simulink library "gps_block_visual"  (R2025b)
settings: Solver=VariableStepAuto  StartTime=0.0  StopTime=10.0  RelTol=1e-3
values from neighbouring files (symbols this model uses):
  GPS = evalin('base', 'GPS')    [test_gps_model.m]
  Sim = evalin('base', 'Sim')    [test_gps_model.m]
settings Model: Creator=Ashwin  LastModifiedBy=Ashwin

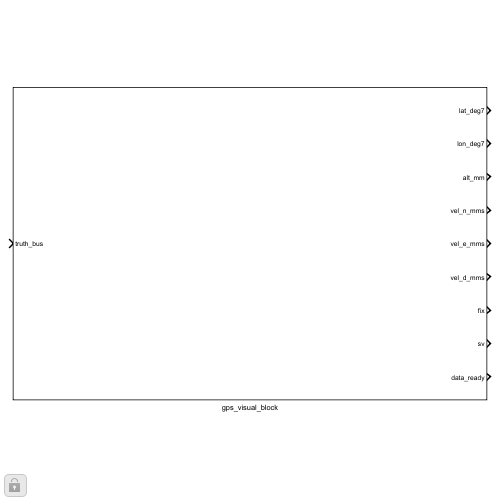
[thumbnail: Simulink's stored preview of the top-level diagram]
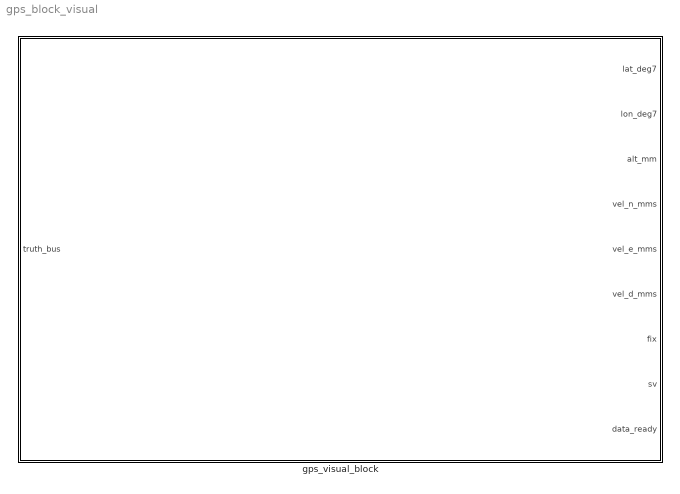
== system gps_block_visual ==
  gps_visual_block : Subsystem

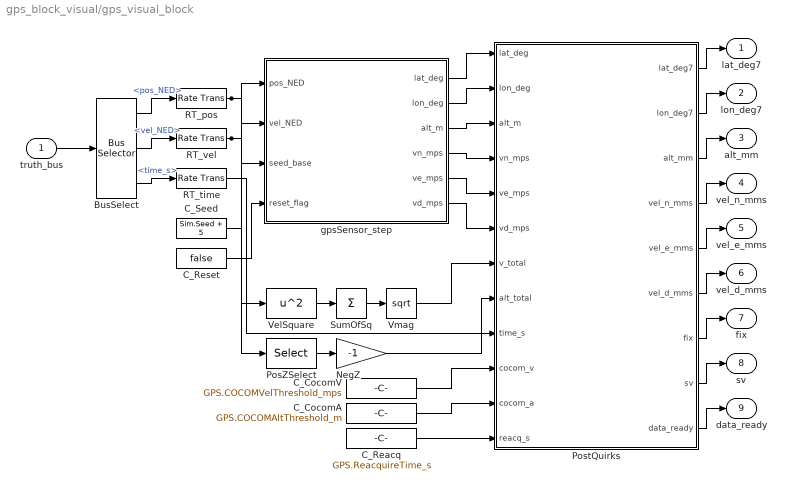
== system gps_block_visual/gps_visual_block ==
  truth_bus : Inport  OutDataTypeStr=Bus: SensorInputBus
  BusSelect : BusSelector  OutputSignals=pos_NED,vel_NED,time_s
  C_CocomA : Constant  Value=GPS.COCOMAltThreshold_m  SampleTime=1/GPS.Rate_Hz
  C_CocomV : Constant  Value=GPS.COCOMVelThreshold_mps  SampleTime=1/GPS.Rate_Hz
  C_Reacq : Constant  Value=GPS.ReacquireTime_s  SampleTime=1/GPS.Rate_Hz
  C_Reset : Constant  Value=false  OutDataTypeStr=boolean  SampleTime=1/GPS.Rate_Hz
  C_Seed : Constant  Value=Sim.Seed + 5  SampleTime=1/GPS.Rate_Hz
  NegZ : Gain  Gain=-1
  PosZSelect : Selector  InputPortWidth=3  IndexOptions=Index vector (dialog)  Indices=3  OutputSizes=1
  PostQuirks : MATLAB Function  TreatAsAtomicUnit=on
  RT_pos : RateTransition  OutPortSampleTime=1/GPS.Rate_Hz
  RT_time : RateTransition  OutPortSampleTime=1/GPS.Rate_Hz
  RT_vel : RateTransition  OutPortSampleTime=1/GPS.Rate_Hz
  SumOfSq : Sum  Inputs=+
  VelSquare : Math  Operator=square
  Vmag : Sqrt
  gpsSensor_step : MATLAB Function  TreatAsAtomicUnit=on
  lat_deg7 : Outport
  lon_deg7 : Outport  Port=2
  alt_mm : Outport  Port=3
  vel_n_mms : Outport  Port=4
  vel_e_mms : Outport  Port=5
  vel_d_mms : Outport  Port=6
  fix : Outport  Port=7
  sv : Outport  Port=8
  data_ready : Outport  Port=9
  wires:
  truth_bus/1 -> BusSelect/1
  BusSelect/1 -> RT_pos/1  "<pos_NED>"
  BusSelect/2 -> RT_vel/1  "<vel_NED>"
  BusSelect/3 -> RT_time/1  "<time_s>"
  RT_pos/1 -> gpsSensor_step/1(pos_NED), PosZSelect/1
  RT_vel/1 -> gpsSensor_step/2(vel_NED), VelSquare/1
  C_Seed/1 -> gpsSensor_step/3(seed_base)
  C_Reset/1 -> gpsSensor_step/4(reset_flag)
  VelSquare/1 -> SumOfSq/1
  SumOfSq/1 -> Vmag/1
  PosZSelect/1 -> NegZ/1
  gpsSensor_step/1(lat_deg) -> PostQuirks/1(lat_deg)
  gpsSensor_step/2(lon_deg) -> PostQuirks/2(lon_deg)
  gpsSensor_step/3(alt_m) -> PostQuirks/3(alt_m)
  gpsSensor_step/4(vn_mps) -> PostQuirks/4(vn_mps)
  gpsSensor_step/5(ve_mps) -> PostQuirks/5(ve_mps)
  gpsSensor_step/6(vd_mps) -> PostQuirks/6(vd_mps)
  Vmag/1 -> PostQuirks/7(v_total)
  NegZ/1 -> PostQuirks/8(alt_total)
  RT_time/1 -> PostQuirks/9(time_s)
  C_CocomV/1 -> PostQuirks/10(cocom_v)
  C_CocomA/1 -> PostQuirks/11(cocom_a)
  C_Reacq/1 -> PostQuirks/12(reacq_s)
  PostQuirks/1(lat_deg7) -> lat_deg7/1
  PostQuirks/2(lon_deg7) -> lon_deg7/1
  PostQuirks/3(alt_mm) -> alt_mm/1
  PostQuirks/4(vel_n_mms) -> vel_n_mms/1
  PostQuirks/5(vel_e_mms) -> vel_e_mms/1
  PostQuirks/6(vel_d_mms) -> vel_d_mms/1
  PostQuirks/7(fix) -> fix/1
  PostQuirks/8(sv) -> sv/1
  PostQuirks/9(data_ready) -> data_ready/1

== matlab function gps_block_visual/gps_visual_block/PostQuirks ==
  data: lat_deg input; lat_deg7 output; lon_deg input; alt_m input; vn_mps input; ve_mps input; vd_mps input; v_total input; alt_total input; time_s input; cocom_v input; cocom_a input; reacq_s input; lon_deg7 output; alt_mm output; vel_n_mms output; vel_e_mms output; vel_d_mms output; fix output; sv output; data_ready output
function [lat_deg7, lon_deg7, alt_mm, vel_n_mms, vel_e_mms, vel_d_mms, fix, sv, data_ready] = fcn(lat_deg, lon_deg, alt_m, vn_mps, ve_mps, vd_mps, v_total, alt_total, time_s, cocom_v, cocom_a, reacq_s)
coder.extrinsic('casper_gps_quirks');
lat_deg7 = int32(0); lon_deg7 = int32(0); alt_mm = int32(0);
vel_n_mms = int32(0); vel_e_mms = int32(0); vel_d_mms = int32(0);
fix = uint8(0); sv = uint8(0); data_ready = false;
[lat_deg7, lon_deg7, alt_mm, vel_n_mms, vel_e_mms, vel_d_mms, fix, sv, data_ready] = casper_gps_quirks(double(lat_deg), double(lon_deg), double(alt_m), double(vn_mps), double(ve_mps), double(vd_mps), double(v_total), double(alt_total), double(time_s), double(cocom_v), double(cocom_a), double(reacq_s));
end

== matlab function gps_block_visual/gps_visual_block/gpsSensor_step ==
  data: pos_NED input; lat_deg output; vel_NED input; seed_base input; reset_flag input; lon_deg output; alt_m output; vn_mps output; ve_mps output; vd_mps output
function [lat_deg, lon_deg, alt_m, vn_mps, ve_mps, vd_mps] = fcn(pos_NED, vel_NED, seed_base, reset_flag)
coder.extrinsic('casper_gps_step_visual');
lat_deg = 0.0; lon_deg = 0.0; alt_m = 0.0;
vn_mps  = 0.0; ve_mps  = 0.0; vd_mps  = 0.0;
[lat_deg, lon_deg, alt_m, vn_mps, ve_mps, vd_mps, ~] = casper_gps_step_visual(pos_NED(:).', vel_NED(:).', double(seed_base), logical(reset_flag));
end
